simulink model "Hover_throttle_baseline"  (R2025b)
settings: Solver=VariableStepAuto  StartTime=0.0  StopTime=10.0  RelTol=1e-3
undefined symbols (not defined in the file): params
settings Model: Creator=samue  LastModifiedBy=samue

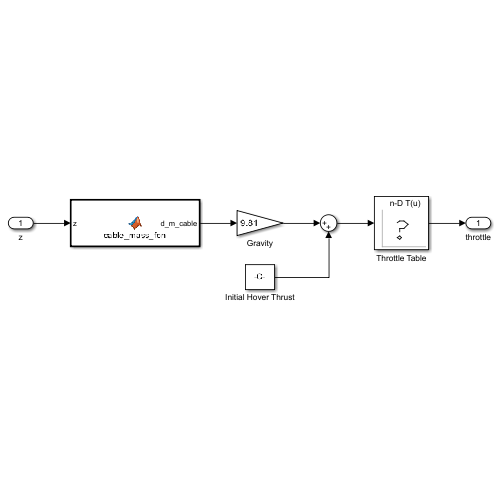
[thumbnail: Simulink's stored preview of the top-level diagram]
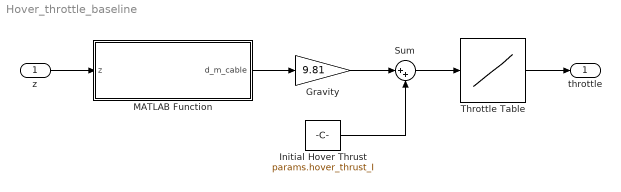
== system Hover_throttle_baseline ==
  z : Inport
  Gravity : Gain  Gain=9.81
  Initial Hover Thrust : Constant  Value=params.hover_thrust_I
  MATLAB Function : MATLAB Function  TreatAsAtomicUnit=on
  Sum : Sum  Inputs=|++
  Throttle Table : Lookup_n-D  NumberOfTableDimensions=1  BreakpointsForDimension1=params.thrust_array  Table=params.throttle_array  InternalRulePriority=Speed  RndMeth=Simplest
  throttle : Outport
  wires:
  Throttle Table/1 -> throttle/1
  z/1 -> MATLAB Function/1(z)
  MATLAB Function/1(d_m_cable) -> Gravity/1
  Gravity/1 -> Sum/1
  Sum/1 -> Throttle Table/1
  Initial Hover Thrust/1 -> Sum/2

== matlab function Hover_throttle_baseline/MATLAB Function ==
  data: d_m_cable output; z input; config parameter
function d_m_cable = cable_mass_fcn(z, config)
% Solves for cable mass based on current height
    % Constants
    cable_length = config.cable_length;
    cable_mass = config.cable_mass;
 
    % Solve for cable mass at current height
    d_m_cable = (cable_mass / cable_length) * z;
end
